simulink model "Flowchart4"  (Simulink 6.0)
settings: Solver=FixedStepDiscrete  StartTime=0.0  StopTime=10.0  RelTol=1e-3
settings Model: Creator=scaife  LastModifiedBy=scaife  ExtModeAutoUpdateStatusClock=off

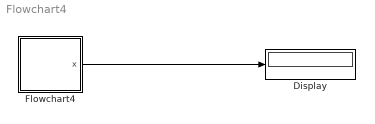
== system Flowchart4 ==
  Display : Display
  Flowchart4 : Stateflow chart
  wires:
  Flowchart4/1(x) -> Display/1

== stateflow chart Flowchart4 ==
  state A
    A -> (junction 4) : {x++;}
  data: x output int32
